simulink model "driftDetect"  (R2018a)
settings: Solver=VariableStepAuto  StartTime=0.0  StopTime=1e4  RelTol=1e-3
libraries: xbsIndex_r4 x79
settings Model: Creator=cganewat18  LastModifiedBy=cganewat18

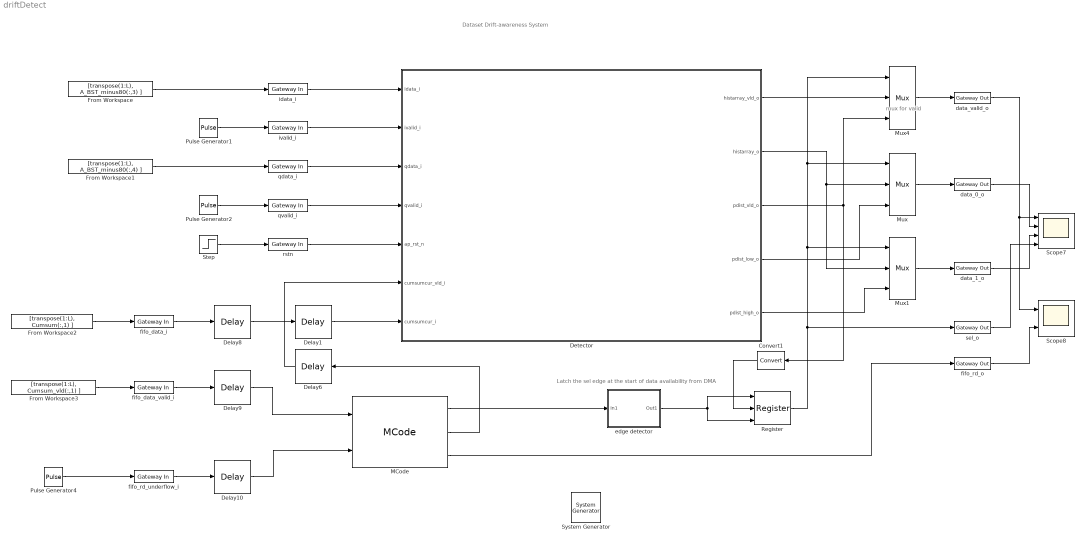
== system driftDetect ==
  note: Dataset Drift-awareness System
  note: mux for valid
  note: Latch the sel edge at the start of data availability from DMA
  " System Generator" : xbsIndex_r4/ System Generator  Tag=genX  xilinxfamily=zynq  part=xc7z020  speed=-1  package=clg484  synthesis_tool=Vivado  clock_wrapper=Clock Enables  directory=./netlist  proj_type=Vivado  Synth_file=Vivado Synthesis Defaults  Impl_file=Vivado Implementation Defaults  testbench=off  simulink_period=1  sysclk_period=8  dcm_input_clock_period=10  incr_netlist=off  trim_vbits=Everywhere in SubSystem  dbl_ovrd=According to Block Masks  core_generation=According to Block Masks  run_coregen=off  deprecated_control=off  eval_field=0  block_type=sysgen
  Convert1 : xbsIndex_r4/Convert  gui_display_data_type=Boolean  arith_type=Boolean  n_bits=1  bin_pt=0  float_type=Single  exp_bits=8  fraction_bits=24  quantization=Truncate  overflow=Wrap  en=off  latency=0  pipeline=off  dbl_ovrd=off  block_type=convert
  Delay{1,6,8..10} (5 alike) : xbsIndex_r4/Delay  rst=off  infoeditControl=Selection of Reset will increase slice count due to use of real FFs and instead of SRLs  en=off  latency=1  reg_retiming=off  dbl_ovrd=off  block_type=delay
  Detector : Subsystem
  From Workspace : FromWorkspace  VariableName=[transpose(1:L), A_BST_minus80(:,3) ]  SampleTime=1  Interpolate=off  OutputAfterFinalValue=Setting to zero
  From Workspace1 : FromWorkspace  VariableName=[transpose(1:L), A_BST_minus80(:,4) ]  SampleTime=1  Interpolate=off  OutputAfterFinalValue=Setting to zero
  From Workspace2 : FromWorkspace  VariableName=[transpose(1:L), Cumsum(:,1) ]  SampleTime=1  Interpolate=off  OutputAfterFinalValue=Setting to zero
  From Workspace3 : FromWorkspace  VariableName=[transpose(1:L), Cumsum_vld(:,1) ]  SampleTime=1  Interpolate=off  OutputAfterFinalValue=Setting to zero
  MCode : xbsIndex_r4/MCode  mfname=state_machine  explicit_period=off  period=1  inputsTable={'boundInpExpr'=>['',''],'inputs'=>['fifo_data_valid_i','fifo_rd_underflow_i']}  outputsTable={'outputs'=>['sel_o','valid_o','fifo_rd_o'],'suppressOut'=>['off','off','off']}  enable_stdout=off  enable_debug=off  suppress_output=on  defparams={}  hide_port_list={}  dbl_ovrd=off  block_type=mcode
  Mux : xbsIndex_r4/Mux  inputs=2  en=off  latency=0  precision=User Defined  arith_type=Unsigned  n_bits=16  bin_pt=0  quantization=Truncate  overflow=Wrap  dbl_ovrd=off  block_type=mux
  Mux1 : xbsIndex_r4/Mux  inputs=2  en=off  latency=0  precision=Full  arith_type=Unsigned  n_bits=16  bin_pt=14  quantization=Truncate  overflow=Wrap  dbl_ovrd=off  block_type=mux
  Mux4 : xbsIndex_r4/Mux  inputs=2  en=off  latency=0  precision=Full  arith_type=Unsigned  n_bits=16  bin_pt=14  quantization=Truncate  overflow=Wrap  dbl_ovrd=off  block_type=mux
  Pulse Generator1 : DiscretePulseGenerator  PulseType=Time based  PulseWidth=50
  Pulse Generator2 : DiscretePulseGenerator  PulseType=Time based  PulseWidth=50
  Pulse Generator4 : DiscretePulseGenerator  PulseType=Time based  Amplitude=0  Period=1  PulseWidth=50
  Register : xbsIndex_r4/Register  init=0  rst=on  en=on  dbl_ovrd=off  block_type=register
  Scope7 : Scope  NumInputPorts=4
      settings: AttributesFormatString=%<Name>
  Scope8 : Scope  NumInputPorts=2
      settings: AttributesFormatString=%<Name>
  Step : Step  SampleTime=0
  data_0_o : xbsIndex_r4/Gateway Out  inherit_from_input=off  hdl_port=on  rows=1  columns=1  UseAsDAC=off  DACChannel='1'  interface=None  automatic_assignment=on  address_offset=hex2dec('00')  intf_name=''  intf_description=''  timing_constraint=None  locs_specified=off  LOCs={}  io_standard={}  block_type=gatewayout
  data_1_o : xbsIndex_r4/Gateway Out  inherit_from_input=off  hdl_port=on  rows=1  columns=1  UseAsDAC=off  DACChannel='1'  interface=None  automatic_assignment=on  address_offset=hex2dec('00')  intf_name=''  intf_description=''  timing_constraint=None  locs_specified=off  LOCs={}  io_standard={}  block_type=gatewayout
  data_valid_o : xbsIndex_r4/Gateway Out  inherit_from_input=off  hdl_port=on  rows=1  columns=1  UseAsDAC=off  DACChannel='1'  interface=None  automatic_assignment=on  address_offset=hex2dec('00')  intf_name=''  intf_description=''  timing_constraint=None  locs_specified=off  LOCs={}  io_standard={}  block_type=gatewayout
  edge detector : Subsystem
  fifo_data_i : xbsIndex_r4/Gateway In  gui_display_data_type=Fixed-point  arith_type=Unsigned  n_bits=32  bin_pt=31  preci_type=Single  exp_width=8  frac_width=24  rows=1  columns=1  quantization="Round  (unbiased: +/- Inf)"  overflow=Saturate  period=1  UseAsADC=off  ADCChannel='1'  interface=None  automatic_assignment=on  address_offset=hex2dec('00')  intf_name=''  intf_description=''  default_value=0  timing_constraint=None  locs_specified=off  LOCs={}  io_standard={}  inherit_from_input=off  hdl_port=on  dbl_ovrd=off  block_type=gatewayin
  fifo_data_valid_i : xbsIndex_r4/Gateway In  gui_display_data_type=Boolean  arith_type=Boolean  n_bits=1  bin_pt=0  preci_type=Single  exp_width=8  frac_width=24  rows=1  columns=1  quantization="Round  (unbiased: +/- Inf)"  overflow=Saturate  period=1  UseAsADC=off  ADCChannel='1'  interface=None  automatic_assignment=on  address_offset=hex2dec('00')  intf_name=''  intf_description=''  default_value=0  timing_constraint=None  locs_specified=off  LOCs={}  io_standard={}  inherit_from_input=off  hdl_port=on  dbl_ovrd=off  block_type=gatewayin
  fifo_rd_o : xbsIndex_r4/Gateway Out  inherit_from_input=off  hdl_port=on  rows=1  columns=1  UseAsDAC=off  DACChannel='1'  interface=None  automatic_assignment=on  address_offset=hex2dec('00')  intf_name=''  intf_description=''  timing_constraint=None  locs_specified=off  LOCs={}  io_standard={}  block_type=gatewayout
  fifo_rd_underflow_i : xbsIndex_r4/Gateway In  gui_display_data_type=Boolean  arith_type=Boolean  n_bits=1  bin_pt=0  preci_type=Single  exp_width=8  frac_width=24  rows=1  columns=1  quantization="Round  (unbiased: +/- Inf)"  overflow=Saturate  period=1  UseAsADC=off  ADCChannel='1'  interface=None  automatic_assignment=on  address_offset=hex2dec('00')  intf_name=''  intf_description=''  default_value=0  timing_constraint=None  locs_specified=off  LOCs={}  io_standard={}  inherit_from_input=off  hdl_port=on  dbl_ovrd=off  block_type=gatewayin
  idata_i : xbsIndex_r4/Gateway In  gui_display_data_type=Fixed-point  arith_type="Signed  (2's comp)"  n_bits=16  bin_pt=0  preci_type=Single  exp_width=8  frac_width=24  rows=1  columns=1  quantization="Round  (unbiased: +/- Inf)"  overflow=Saturate  period=1  UseAsADC=off  ADCChannel='1'  interface=None  automatic_assignment=on  address_offset=hex2dec('00')  intf_name=''  intf_description='Idata'  default_value=0  timing_constraint=None  locs_specified=off  LOCs={}  io_standard={}  inherit_from_input=off  hdl_port=on  dbl_ovrd=off  block_type=gatewayin
  ivalid_i : xbsIndex_r4/Gateway In  gui_display_data_type=Boolean  arith_type=Boolean  n_bits=16  bin_pt=0  preci_type=Single  exp_width=8  frac_width=24  rows=1  columns=1  quantization="Round  (unbiased: +/- Inf)"  overflow=Saturate  period=1  UseAsADC=off  ADCChannel='1'  interface=None  automatic_assignment=on  address_offset=hex2dec('00')  intf_name=''  intf_description='qdata'  default_value=0  timing_constraint=None  locs_specified=off  LOCs={}  io_standard={}  inherit_from_input=off  hdl_port=on  dbl_ovrd=off  block_type=gatewayin
  qdata_i : xbsIndex_r4/Gateway In  gui_display_data_type=Fixed-point  arith_type="Signed  (2's comp)"  n_bits=16  bin_pt=0  preci_type=Single  exp_width=8  frac_width=24  rows=1  columns=1  quantization="Round  (unbiased: +/- Inf)"  overflow=Saturate  period=1  UseAsADC=off  ADCChannel='1'  interface=None  automatic_assignment=on  address_offset=hex2dec('00')  intf_name=''  intf_description='qdata'  default_value=0  timing_constraint=None  locs_specified=off  LOCs={}  io_standard={}  inherit_from_input=off  hdl_port=on  dbl_ovrd=off  block_type=gatewayin
  qvalid_i : xbsIndex_r4/Gateway In  gui_display_data_type=Boolean  arith_type=Boolean  n_bits=16  bin_pt=0  preci_type=Single  exp_width=8  frac_width=24  rows=1  columns=1  quantization="Round  (unbiased: +/- Inf)"  overflow=Saturate  period=1  UseAsADC=off  ADCChannel='1'  interface=None  automatic_assignment=on  address_offset=hex2dec('00')  intf_name=''  intf_description='qdata'  default_value=0  timing_constraint=None  locs_specified=off  LOCs={}  io_standard={}  inherit_from_input=off  hdl_port=on  dbl_ovrd=off  block_type=gatewayin
  rstn : xbsIndex_r4/Gateway In  gui_display_data_type=Boolean  arith_type=Boolean  n_bits=1  bin_pt=0  preci_type=Single  exp_width=8  frac_width=24  rows=1  columns=1  quantization="Round  (unbiased: +/- Inf)"  overflow=Saturate  period=1  UseAsADC=off  ADCChannel='1'  interface=None  automatic_assignment=on  address_offset=hex2dec('00')  intf_name=''  intf_description='qdata'  default_value=0  timing_constraint=None  locs_specified=off  LOCs={}  io_standard={}  inherit_from_input=off  hdl_port=on  dbl_ovrd=off  block_type=gatewayin
  sel_o : xbsIndex_r4/Gateway Out  inherit_from_input=off  hdl_port=on  rows=1  columns=1  UseAsDAC=off  DACChannel='1'  interface=None  automatic_assignment=on  address_offset=hex2dec('00')  intf_name=''  intf_description=''  timing_constraint=None  locs_specified=off  LOCs={}  io_standard={}  block_type=gatewayout
  wires:
  Convert1/1 -> Register/2
  Delay6/1 -> Detector/6(cumsumcur_vld_i)
  sel_o/1 -> Scope7/4
  fifo_rd_underflow_i/1 -> Delay10/1
  Delay1/1 -> Detector/7(cumsumcur_i)
  Delay10/1 -> MCode/2
  data_0_o/1 -> Scope7/2
  Mux1/1 -> data_1_o/1
  MCode/2 -> Delay6/1
  fifo_rd_o/1 -> Scope8/2
  data_valid_o/1 -> Scope8/1, Scope7/1
  idata_i/1 -> Detector/1(idata_i)
  Delay8/1 -> Delay1/1
  From Workspace2/1 -> fifo_data_i/1
  fifo_data_valid_i/1 -> Delay9/1
  From Workspace3/1 -> fifo_data_valid_i/1
  Detector/1(histarray_vld_o) -> Mux4/2
  Detector/3(pdist_vld_o) -> Mux4/3, Convert1/1
  MCode/1 -> edge detector/1(In1)
  edge detector/1(Out1) -> Register/1, Register/3
  Mux/1 -> data_0_o/1
  Delay9/1 -> MCode/1
  qdata_i/1 -> Detector/3(qdata_i)
  MCode/3 -> fifo_rd_o/1
  Detector/4(pdist_low_o) -> Mux/3
  qvalid_i/1 -> Detector/4(qvalid_i)
  rstn/1 -> Detector/5(ap_rst_n)
  Mux4/1 -> data_valid_o/1
  Register/1 -> sel_o/1, Mux1/1, Mux/1, Mux4/1
  Detector/5(pdist_high_o) -> Mux1/3
  ivalid_i/1 -> Detector/2(ivalid_i)
  Step/1 -> rstn/1
  Pulse Generator4/1 -> fifo_rd_underflow_i/1
  From Workspace1/1 -> qdata_i/1
  fifo_data_i/1 -> Delay8/1
  From Workspace/1 -> idata_i/1
  Pulse Generator2/1 -> qvalid_i/1
  data_1_o/1 -> Scope7/3
  Detector/2(histarray_o) -> Mux1/2, Mux/2
  Pulse Generator1/1 -> ivalid_i/1

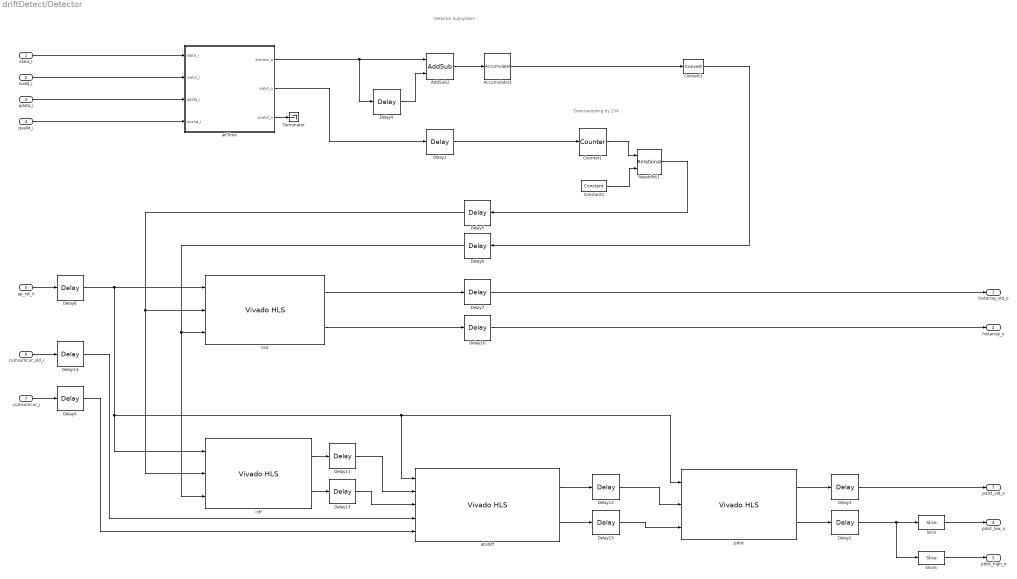
== system driftDetect/Detector ==
  note: Detector Subsystem
  note: Downsampling by 256
  idata_i : Inport
  ivalid_i : Inport  Port=2
  qdata_i : Inport  Port=3
  qvalid_i : Inport  Port=4
  ap_rst_n : Inport  Port=5
  cumsumcur_vld_i : Inport  Port=6
  cumsumcur_i : Inport  Port=7
  Accumulator1 : xbsIndex_r4/Accumulator  operation=Add  n_bits=16  overflow=Wrap  scale=1  rst=off  hasbypass=off  infoeditControl=reset for floating point data type must be asserted for a minimum of 2 cycles  en=off  latency=1  msb_inp=100  msb=100  lsb=-100  use_behavioral_HDL=on  implementation=Fabric  dbl_ovrd=off  block_type=accum
  AddSub2 : xbsIndex_r4/AddSub  mode=Subtraction  use_carryin=off  use_carryout=off  en=off  latency=1  precision=Full  arith_type=Unsigned  n_bits=16  bin_pt=14  quantization=Truncate  overflow=Wrap  use_behavioral_HDL=off  hw_selection=Fabric  pipelined=off  dbl_ovrd=off  block_type=addsub
  Constant1 : xbsIndex_r4/Constant  const=255  gui_display_data_type=Fixed-point  arith_type=Unsigned  n_bits=13  bin_pt=0  preci_type=Single  exp_width=8  frac_width=24  explicit_period=off  period=1  equ=P=C  opselect=C  inp2=PCIN>>17  opr=+  inp1=P  carry=CIN  dbl_ovrd=off  block_type=constant
  Convert1 : xbsIndex_r4/Convert  gui_display_data_type=Fixed-point  arith_type=Unsigned  n_bits=16  bin_pt=0  float_type=Single  exp_bits=8  fraction_bits=24  quantization=Truncate  overflow=Wrap  en=off  latency=0  pipeline=off  dbl_ovrd=off  block_type=convert
  Counter1 : xbsIndex_r4/Counter  cnt_type=Free Running  cnt_to=1000  operation=Up  start_count=0  cnt_by_val=1  arith_type=Unsigned  n_bits=8  bin_pt=0  load_pin=off  rst=off  en=on  explicit_period=on  period=1  use_behavioral_HDL=off  implementation=Fabric  dbl_ovrd=off  block_type=counter
  Delay1 : xbsIndex_r4/Delay  rst=off  infoeditControl=Selection of Reset will increase slice count due to use of real FFs and instead of SRLs  en=off  latency=2  reg_retiming=off  dbl_ovrd=off  block_type=delay
  Delay{2..3,5..15} (13 alike) : xbsIndex_r4/Delay  rst=off  infoeditControl=Selection of Reset will increase slice count due to use of real FFs and instead of SRLs  en=off  latency=1  reg_retiming=off  dbl_ovrd=off  block_type=delay
  Delay4 : xbsIndex_r4/Delay  rst=off  infoeditControl=Selection of Reset will increase slice count due to use of real FFs and instead of SRLs  en=off  latency=10000  reg_retiming=off  dbl_ovrd=off  block_type=delay
  Resetifhit1 : xbsIndex_r4/Relational  mode=a=b  op_type=Bool  en=off  latency=0  dbl_ovrd=off  block_type=relational
  Slice : xbsIndex_r4/Slice  nbits=1  boolean_output=off  mode=Two Bit Locations  bit1=15  base1=LSB of Input  bit0=0  base0=LSB of Input  dbl_ovrd=off  block_type=slice
  Slice1 : xbsIndex_r4/Slice  nbits=1  boolean_output=off  mode=Two Bit Locations  bit1=31  base1=LSB of Input  bit0=16  base0=LSB of Input  dbl_ovrd=off  block_type=slice
  Terminator : Terminator
  absdiff : xbsIndex_r4/Vivado HLS  anytable='../HLS/absdiff/solution1'  fast_sim=off  display_datatype=on  rate_propagation_method=Simulink system period  model_file_path=''  latency=1  block_type=hls
      settings: infoedit=This block allows including C,C++ and SystemC source files in System Generator for DSP designs.
  airTime : Subsystem
  cdf : xbsIndex_r4/Vivado HLS  anytable='../HLS/cdf/solution1'  fast_sim=off  display_datatype=on  rate_propagation_method=Simulink system period  model_file_path=''  latency=1  block_type=hls
      settings: infoedit=This block allows including C,C++ and SystemC source files in System Generator for DSP designs.
  hist : xbsIndex_r4/Vivado HLS  anytable='../HLS/hist/solution1'  fast_sim=off  display_datatype=on  rate_propagation_method=Simulink system period  model_file_path=''  latency=1  block_type=hls
      settings: infoedit=This block allows including C,C++ and SystemC source files in System Generator for DSP designs.
  pdist : xbsIndex_r4/Vivado HLS  anytable='../HLS/pdist/solution1'  fast_sim=off  display_datatype=on  rate_propagation_method=Simulink system period  model_file_path=''  latency=1  block_type=hls
      settings: infoedit=This block allows including C,C++ and SystemC source files in System Generator for DSP designs.
  histarray_vld_o : Outport
  histarray_o : Outport  Port=2
  pdist_vld_o : Outport  Port=3
  pdist_low_o : Outport  Port=4
  pdist_high_o : Outport  Port=5
  wires:
  AddSub2/1 -> Accumulator1/1
  airTime/1(airtime_o) -> Delay4/1, AddSub2/1
  Resetifhit1/1 -> Delay5/1
  ivalid_i/1 -> airTime/2(ivalid_i)
  Counter1/1 -> Resetifhit1/1
  airTime/3(qvalid_o) -> Terminator/1
  hist/2 -> Delay10/1
  qvalid_i/1 -> airTime/4(qvalid_i)
  Delay15/1 -> pdist/3
  Delay9/1 -> absdiff/5
  Delay8/1 -> hist/1, cdf/1, pdist/1, absdiff/1
  Delay11/1 -> absdiff/2
  airTime/2(ivalid_o) -> Delay1/1
  Constant1/1 -> Resetifhit1/2
  Delay6/1 -> cdf/3, hist/3
  absdiff/1 -> Delay12/1
  cumsumcur_vld_i/1 -> Delay14/1
  cdf/1 -> Delay11/1
  Delay12/1 -> pdist/2
  cdf/2 -> Delay13/1
  Delay1/1 -> Counter1/1
  Delay14/1 -> absdiff/4
  absdiff/2 -> Delay15/1
  Convert1/1 -> Delay6/1
  pdist/1 -> Delay3/1
  Delay4/1 -> AddSub2/2
  Delay10/1 -> histarray_o/1
  Delay13/1 -> absdiff/3
  Delay7/1 -> histarray_vld_o/1
  Delay5/1 -> cdf/2, hist/2
  Accumulator1/1 -> Convert1/1
  hist/1 -> Delay7/1
  pdist/2 -> Delay2/1
  qdata_i/1 -> airTime/3(qdata_i)
  Slice1/1 -> pdist_high_o/1
  cumsumcur_i/1 -> Delay9/1
  Slice/1 -> pdist_low_o/1
  idata_i/1 -> airTime/1(idata_i)
  ap_rst_n/1 -> Delay8/1
  Delay3/1 -> pdist_vld_o/1
  Delay2/1 -> Slice/1, Slice1/1

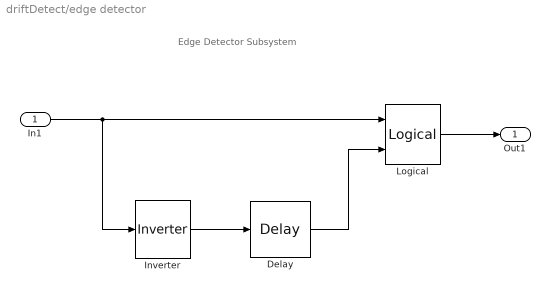
== system driftDetect/edge detector ==
  note: Edge Detector Subsystem
  In1 : Inport
  Delay : xbsIndex_r4/Delay  rst=off  infoeditControl=Selection of Reset will increase slice count due to use of real FFs and instead of SRLs  en=off  latency=1  reg_retiming=off  dbl_ovrd=off  block_type=delay
  Inverter : xbsIndex_r4/Inverter  en=off  latency=0  dbl_ovrd=off  block_type=inv
  Logical : xbsIndex_r4/Logical  logical_function=AND  inputs=2  en=off  latency=0  precision=Full  arith_type=Unsigned  n_bits=16  bin_pt=0  align_bp=on  dbl_ovrd=off  block_type=logical
  Out1 : Outport
  wires:
  Delay/1 -> Logical/2
  Logical/1 -> Out1/1
  In1/1 -> Inverter/1, Logical/1
  Inverter/1 -> Delay/1

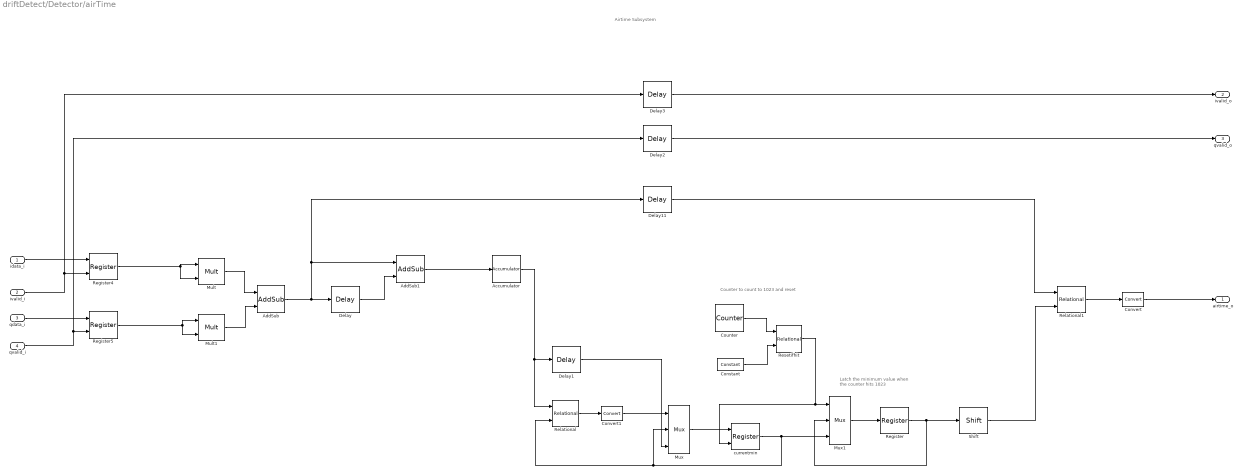
== system driftDetect/Detector/airTime ==
  note: Airtime Subsystem
  note: Counter to count to 1023 and reset
  note: Latch the minimum value when
      | the counter hits 1023
  idata_i : Inport
  ivalid_i : Inport  Port=2
  qdata_i : Inport  Port=3
  qvalid_i : Inport  Port=4
  Accumulator : xbsIndex_r4/Accumulator  operation=Add  n_bits=32  overflow=Wrap  scale=1  rst=off  hasbypass=off  infoeditControl=reset for floating point data type must be asserted for a minimum of 2 cycles  en=off  latency=1  msb_inp=100  msb=100  lsb=-100  use_behavioral_HDL=on  implementation=Fabric  dbl_ovrd=off  block_type=accum
  AddSub : xbsIndex_r4/AddSub  mode=Addition  use_carryin=off  use_carryout=off  en=off  latency=1  precision=Full  arith_type=Unsigned  n_bits=16  bin_pt=14  quantization=Truncate  overflow=Wrap  use_behavioral_HDL=off  hw_selection=Fabric  pipelined=off  dbl_ovrd=off  block_type=addsub
  AddSub1 : xbsIndex_r4/AddSub  mode=Subtraction  use_carryin=off  use_carryout=off  en=off  latency=1  precision=Full  arith_type=Unsigned  n_bits=16  bin_pt=14  quantization=Truncate  overflow=Wrap  use_behavioral_HDL=off  hw_selection=Fabric  pipelined=off  dbl_ovrd=off  block_type=addsub
  Constant : xbsIndex_r4/Constant  const=1023  gui_display_data_type=Fixed-point  arith_type=Unsigned  n_bits=10  bin_pt=0  preci_type=Single  exp_width=8  frac_width=24  explicit_period=off  period=1  equ=P=C  opselect=C  inp2=PCIN>>17  opr=+  inp1=P  carry=CIN  dbl_ovrd=off  block_type=constant
  Convert : xbsIndex_r4/Convert  gui_display_data_type=Fixed-point  arith_type=Unsigned  n_bits=1  bin_pt=0  float_type=Single  exp_bits=8  fraction_bits=24  quantization=Truncate  overflow=Wrap  en=off  latency=0  pipeline=off  dbl_ovrd=off  block_type=convert
  Convert1 : xbsIndex_r4/Convert  gui_display_data_type=Fixed-point  arith_type=Unsigned  n_bits=1  bin_pt=0  float_type=Single  exp_bits=8  fraction_bits=24  quantization=Truncate  overflow=Wrap  en=off  latency=0  pipeline=off  dbl_ovrd=off  block_type=convert
  Counter : xbsIndex_r4/Counter  cnt_type=Free Running  cnt_to=1000  operation=Up  start_count=0  cnt_by_val=1  arith_type=Unsigned  n_bits=10  bin_pt=0  load_pin=off  rst=off  en=off  explicit_period=on  period=1  use_behavioral_HDL=off  implementation=Fabric  dbl_ovrd=off  block_type=counter
  Delay : xbsIndex_r4/Delay  rst=off  infoeditControl=Selection of Reset will increase slice count due to use of real FFs and instead of SRLs  en=off  latency=64  reg_retiming=off  dbl_ovrd=off  block_type=delay
  Delay1 : xbsIndex_r4/Delay  rst=off  infoeditControl=Selection of Reset will increase slice count due to use of real FFs and instead of SRLs  en=off  latency=1  reg_retiming=off  dbl_ovrd=off  block_type=delay
  Delay11 : xbsIndex_r4/Delay  rst=off  infoeditControl=Selection of Reset will increase slice count due to use of real FFs and instead of SRLs  en=off  latency=6  reg_retiming=off  dbl_ovrd=off  block_type=delay
  Delay2 : xbsIndex_r4/Delay  rst=off  infoeditControl=Selection of Reset will increase slice count due to use of real FFs and instead of SRLs  en=off  latency=12  reg_retiming=off  dbl_ovrd=off  block_type=delay
  Delay3 : xbsIndex_r4/Delay  rst=off  infoeditControl=Selection of Reset will increase slice count due to use of real FFs and instead of SRLs  en=off  latency=12  reg_retiming=off  dbl_ovrd=off  block_type=delay
  Mult : xbsIndex_r4/Mult  precision=Full  arith_type="Signed  (2's comp)"  n_bits=16  bin_pt=14  quantization=Truncate  overflow=Wrap  en=off  latency=3  use_behavioral_HDL=off  opt=Speed  use_embedded=on  optimum_pipeline=off  pipeline=on  dbl_ovrd=off  use_rpm=on  placement_style=Triangular  block_type=mult
  Mult1 : xbsIndex_r4/Mult  precision=Full  arith_type="Signed  (2's comp)"  n_bits=16  bin_pt=14  quantization=Truncate  overflow=Wrap  en=off  latency=3  use_behavioral_HDL=off  opt=Speed  use_embedded=on  optimum_pipeline=off  pipeline=on  dbl_ovrd=off  use_rpm=on  placement_style=Triangular  block_type=mult
  Mux : xbsIndex_r4/Mux  inputs=2  en=off  latency=0  precision=Full  arith_type=Unsigned  n_bits=16  bin_pt=14  quantization=Truncate  overflow=Wrap  dbl_ovrd=off  block_type=mux
  Mux1 : xbsIndex_r4/Mux  inputs=2  en=off  latency=0  precision=Full  arith_type=Unsigned  n_bits=16  bin_pt=14  quantization=Truncate  overflow=Wrap  dbl_ovrd=off  block_type=mux
  Register : xbsIndex_r4/Register  init=2e8  rst=off  en=off  dbl_ovrd=off  block_type=register
  Register4 : xbsIndex_r4/Register  init=0  rst=off  en=on  dbl_ovrd=off  block_type=register
  Register5 : xbsIndex_r4/Register  init=0  rst=off  en=on  dbl_ovrd=off  block_type=register
  Relational : xbsIndex_r4/Relational  mode=a<b  op_type=Bool  en=off  latency=1  dbl_ovrd=off  block_type=relational
  Relational1 : xbsIndex_r4/Relational  mode=a>b  op_type=Bool  en=off  latency=1  dbl_ovrd=off  block_type=relational
  Resetifhit : xbsIndex_r4/Relational  mode=a=b  op_type=Bool  en=off  latency=0  dbl_ovrd=off  block_type=relational
  Shift : xbsIndex_r4/Shift  Description=Divide by the moving average filter size. Here 64. So, have to right shift by 6 bits.  shift_dir=Right  shift_bits=2  en=off  latency=1  precision=Full  arith_type="Signed  (2's comp)"  n_bits=16  bin_pt=14  quantization=Truncate  overflow=Wrap  dbl_ovrd=off  block_type=shift
  currentmin : xbsIndex_r4/Register  init=2e8  rst=on  en=off  dbl_ovrd=off  block_type=register
  airtime_o : Outport
  ivalid_o : Outport  Port=2
  qvalid_o : Outport  Port=3
  wires:
  Register/1 -> Mux1/2, Shift/1
  Delay11/1 -> Relational1/1
  AddSub/1 -> Delay/1, Delay11/1, AddSub1/1
  idata_i/1 -> Register4/1
  Counter/1 -> Resetifhit/1
  Relational/1 -> Convert1/1
  Constant/1 -> Resetifhit/2
  Register4/1 -> Mult/2, Mult/1
  Register5/1 -> Mult1/2, Mult1/1
  qvalid_i/1 -> Delay2/1, Register5/2
  ivalid_i/1 -> Delay3/1, Register4/2
  Mult1/1 -> AddSub/2
  Accumulator/1 -> Relational/1, Delay1/1
  currentmin/1 -> Relational/2, Mux/2, Mux1/3
  Mux1/1 -> Register/1
  Relational1/1 -> Convert/1
  Resetifhit/1 -> currentmin/2, Mux1/1
  Delay1/1 -> Mux/3
  Shift/1 -> Relational1/2
  Convert1/1 -> Mux/1
  qdata_i/1 -> Register5/1
  AddSub1/1 -> Accumulator/1
  Mult/1 -> AddSub/1
  Mux/1 -> currentmin/1
  Delay2/1 -> qvalid_o/1
  Delay/1 -> AddSub1/2
  Delay3/1 -> ivalid_o/1
  Convert/1 -> airtime_o/1
